simulink library "myAlgorithmLib"  (R2017b)
settings: Solver=VariableStepAuto  StartTime=0.0  StopTime=10.0  RelTol=1e-3
values from neighbouring files (symbols this model uses):
  ctrlParam1 = 2    [myPreloadScript.m]
  ctrlParam2 = 3.5    [myPreloadScript.m]
  sampleTimeFast = 0.2    [myPreloadScript.m]
settings Model: Creator=scastro  LastModifiedBy=scastro

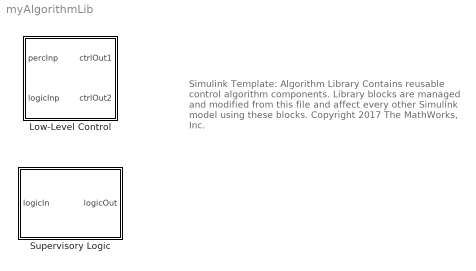
== system myAlgorithmLib ==
  note: Simulink Template: Algorithm Library
      |
      | Contains reusable control algorithm components.
      |
      | Library blocks are managed and modified from this file and affect every other Simulink model using these blocks.
      |
      | Copyright 2017 The MathWorks, Inc.
  Low-Level Control : Subsystem  mask(Low-Level Control Template){k1=ctrlParam1, k2=ctrlParam2, Ts=sampleTimeFast}
      mask prompts: k1 "Parameter 1"; k2 "Parameter 2"; Ts "Sample Time"
      mask help:
      | This block accepts two mask dialog parameters as controller gains.
      |
      | Right-click this block and select "Mask > Look Under Mask" to see the contents of the block.
  Supervisory Logic : Stateflow chart  TreatAsAtomicUnit=on

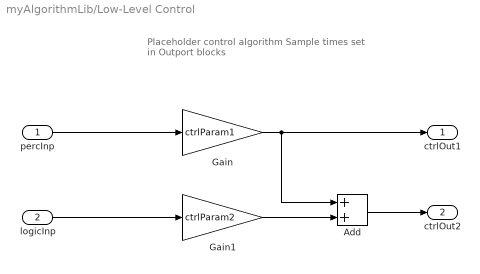
== system myAlgorithmLib/Low-Level Control ==
  note: Placeholder control algorithm
      |
      | Sample times set in Outport blocks
  percInp : Inport
  logicInp : Inport  Port=2
  Add : Sum
  Gain : Gain  Gain=ctrlParam1
  Gain1 : Gain  Gain=ctrlParam2
  ctrlOut1 : Outport  SampleTime=Ts
      settings: AttributesFormatString=Sample time: %<SampleTime>
  ctrlOut2 : Outport  Port=2  SampleTime=Ts
      settings: AttributesFormatString=Sample time: %<SampleTime>
  wires:
  logicInp/1 -> Gain1/1
  percInp/1 -> Gain/1
  Gain/1 -> Add/1, ctrlOut1/1
  Add/1 -> ctrlOut2/1
  Gain1/1 -> Add/2

== stateflow chart myAlgorithmLib/Supervisory Logic ==
  state ModeA
    % First operating mode
    entry:
    logicOut = 1;
  state ModeB
    % Second operating mode
    entry:
    logicOut = -1;
  (default) -> ModeA
  ModeB -> ModeA : [logicIn < 0]
  ModeA -> ModeB : [logicIn >= 0]
  data: logicIn input; logicOut output
